simulink model "CalibrationMotorbike_v2"  (R2020b)
settings: Solver=FixedStepDiscrete  StartTime=0.0  StopTime=inf  FixedStep=0.01  RelTol=1e-3  EnableMultiTasking=on
undefined symbols (not defined in the file or in its folder): fdesignblkfcn, gcbh
libraries: dspstat3 x11, dsparch4 x3, simulink x2, dspswit3 x1
(part 2 of 2)

== system CalibrationMotorbike_v2/Butterworth2nd9 ==
  cutOff-Freq : Inport
  U(t) : Inport  Port=2
  samplingTime : Inport  Port=3
  Add : Sum  Inputs=+++
  Add1 : Sum  Inputs=+-
  Add2 : Sum
  Add3 : Sum  Inputs=+-+
  Add4 : Sum
  Add5 : Sum  Inputs=+++
  Divide : Product  Inputs=*/
  Divide1 : Product  Inputs=*/
  Gain : Gain  Gain=2
  Gain1 : Gain  Gain=sqrt(2)
  Gain2 : Gain  Gain=2
  Gain3 : Gain  Gain=-2
  Product{,1..5,7..9} (9 alike) : Product  RndMeth=Zero
  Unit Delay{,1,3..4} (4 alike) : UnitDelay  SampleTime=-1  HasFrameUpgradeWarning=on
  const : Constant  Value=2*pi
  const3 : Constant  Value=2
  Y(t) : Outport  VectorParamsAs1DForOutWhenUnconnected=off
  wires:
  U(t)/1 -> Product1/2, Unit Delay/1
  Product/1 -> Product1/1, Product3/1, Product2/1, Gain/1, Add3/3, Add5/3
  Unit Delay/1 -> Unit Delay1/1, Gain2/1
  Unit Delay1/1 -> Product3/2
  Product1/1 -> Add/1
  Product2/1 -> Add/2
  Product3/1 -> Add/3
  Add/1 -> Add1/1
  Divide/1 -> Unit Delay3/1, Y(t)/1
  Product4/1 -> Add3/1, Add5/1, Gain3/1
  Gain/1 -> Add2/1
  Unit Delay3/1 -> Product7/2, Unit Delay4/1
  Add2/1 -> Product7/1
  Gain1/1 -> Product8/1
  Product8/1 -> Add3/2, Add5/2
  Unit Delay4/1 -> Product9/2
  Add3/1 -> Product9/1
  Product9/1 -> Add4/2
  Product7/1 -> Add4/1
  Add4/1 -> Add1/2
  Add1/1 -> Divide/1
  Add5/1 -> Divide/2
  Gain2/1 -> Product2/2
  Gain3/1 -> Add2/2
  Product5/1 -> Product/1, Product/2, Product8/2
  const/1 -> Product5/1
  cutOff-Freq/1 -> Product5/2
  const3/1 -> Divide1/1
  samplingTime/1 -> Divide1/2
  Divide1/1 -> Gain1/1, Product4/2, Product4/1

== system CalibrationMotorbike_v2/Double-Click Button to set current folder ==

== system CalibrationMotorbike_v2/Simulink Function ==
  Gravity_2_RotMatrix : TriggerPort  TriggerType=function-call  IsSimulinkFunction=on  FunctionName=Gravity_2_RotMatrix  FunctionVisibility=scoped  VariantControl=(inherit)
  Gravity_2_RotMatrixMat : MATLAB Function  TreatAsAtomicUnit=on
  gravity : ArgIn  DisableCoverage=on  OutDataTypeStr=single  PortDimensions=4  ArgumentName=gravity
  rot_Matrix : ArgOut  DisableCoverage=on  OutDataTypeStr=single  PortDimensions=[3 3]  ArgumentName=rot_Matrix
  wires:
  gravity/1 -> Gravity_2_RotMatrixMat/1(gravity)
  Gravity_2_RotMatrixMat/1(A) -> rot_Matrix/1

== system CalibrationMotorbike_v2/SmartACCFilter1 ==
  ACC_In : Inport
  Moving Average2 : dspstat3/Moving Average  Method=Sliding window  ForgettingFactorPort=off  SpecifyWindowLength=on  WindowLength=40  ForgettingFactor=0.9  SimulateUsing=Code generation
  Moving Standard Deviation2 : dspstat3/Moving Standard Deviation  Method=Sliding window  ForgettingFactorPort=off  SpecifyWindowLength=on  WindowLength=40  ForgettingFactor=0.9  SimulateUsing=Code generation
      settings: SourceProductBaseCode=DS
  SmartFilter2 : MATLAB Function  TreatAsAtomicUnit=on
  accSf_mg_SmartFilter : Outport
  accSf_mg_SmartFilter_k : Outport  Port=2
  accSf_mg_Average20 : Outport  Port=3
  accSf_mg_Std20 : Outport  Port=4
  wires:
  SmartFilter2/2(k_out) -> accSf_mg_SmartFilter_k/1
  SmartFilter2/1(y_out) -> accSf_mg_SmartFilter/1
  Moving Average2/1 -> accSf_mg_Average20/1, SmartFilter2/1(x_mean)  "accSfXmg_Average20"
  Moving Standard Deviation2/1 -> SmartFilter2/2(x_std), accSf_mg_Std20/1
  ACC_In/1 -> Moving Average2/1, Moving Standard Deviation2/1

== system CalibrationMotorbike_v2/SmartACCFilter2 ==
  note: Smart Filtering depending on current noise/motion
      |
      | Low-Noise/Motion	-> fast signal following
      | High-Noise/Motion	-> high filtering (=slow following)
  ACC_In : Inport
  Moving Average2 : dspstat3/Moving Average  Method=Sliding window  ForgettingFactorPort=off  SpecifyWindowLength=on  WindowLength=40  ForgettingFactor=0.9  SimulateUsing=Code generation
  Moving Standard Deviation2 : dspstat3/Moving Standard Deviation  Method=Sliding window  ForgettingFactorPort=off  SpecifyWindowLength=on  WindowLength=40  ForgettingFactor=0.9  SimulateUsing=Code generation
      settings: SourceProductBaseCode=DS
  SmartFilter2 : MATLAB Function  TreatAsAtomicUnit=on
  accSf_mg_SmartFilter : Outport
  accSf_mg_SmartFilter_k : Outport  Port=2
  accSf_mg_Average20 : Outport  Port=3
  accSf_mg_Std20 : Outport  Port=4
  wires:
  ACC_In/1 -> Moving Standard Deviation2/1, Moving Average2/1
  Moving Standard Deviation2/1 -> accSf_mg_Std20/1, SmartFilter2/2(x_std)
  Moving Average2/1 -> SmartFilter2/1(x_mean), accSf_mg_Average20/1  "accSfXmg_Average20"
  SmartFilter2/1(y_out) -> accSf_mg_SmartFilter/1
  SmartFilter2/2(k_out) -> accSf_mg_SmartFilter_k/1

== system CalibrationMotorbike_v2/SmartACCFilter3 ==
  ACC_In : Inport
  Moving Average2 : dspstat3/Moving Average  Method=Sliding window  ForgettingFactorPort=off  SpecifyWindowLength=on  WindowLength=40  ForgettingFactor=0.9  SimulateUsing=Code generation
  Moving Standard Deviation2 : dspstat3/Moving Standard Deviation  Method=Sliding window  ForgettingFactorPort=off  SpecifyWindowLength=on  WindowLength=40  ForgettingFactor=0.9  SimulateUsing=Code generation
      settings: SourceProductBaseCode=DS
  SmartFilter2 : MATLAB Function  TreatAsAtomicUnit=on
  accSf_mg_SmartFilter : Outport
  accSf_mg_SmartFilter_k : Outport  Port=2
  accSf_mg_Average20 : Outport  Port=3
  accSf_mg_Std20 : Outport  Port=4
  wires:
  ACC_In/1 -> Moving Standard Deviation2/1, Moving Average2/1
  Moving Standard Deviation2/1 -> accSf_mg_Std20/1, SmartFilter2/2(x_std)
  Moving Average2/1 -> SmartFilter2/1(x_mean), accSf_mg_Average20/1  "accSfXmg_Average20"
  SmartFilter2/1(y_out) -> accSf_mg_SmartFilter/1
  SmartFilter2/2(k_out) -> accSf_mg_SmartFilter_k/1

== matlab function CalibrationMotorbike_v2/SmartACCFilter1/SmartFilter2 ==
  data: x_mean input; y_out output; x_std input; k_out output
function [y_out,k_out]= fcn(x_mean, x_std)
    persistent y;
    persistent k;

    k_max   =  5;
    k_min   =  0.001;
    k_filter =  0.001;
    std_min =  1000;
    std_max =  2000;
    
    % Initialisation of internal Buffers on Startup
    if isempty(y)        
            y = double(x_mean);
            k = k_max;
    end
    
    
    % Adapt k Lowpass in dependancy of Standard daviation (low noise = const. Riding = faster filter)      
    k_in = k_min;
    if (x_std<std_min)
        k_in = double(k_max);
    elseif (x_std<std_max)
        k_in = double( (((k_min-k_max)/(std_max-std_min))*(x_std-std_min)+k_max));
    else
        k_in = double(k_min);
    end

    % Smoothen k filter to avoid fast k-changes in small low-noise
    % sequences
    % if k is smaller/slower (due to noise in signal) always reduce k fast
    if (k_in > k)
        k = k_filter*k_in + (1-k_filter) * k;
    else
        k = k_in;
    end
    
    %lowpass of Rawdata
    y = double(((1000-k)*y + k * x_mean)/1000);

    k_out = k;
    y_out = y;
end

== matlab function CalibrationMotorbike_v2/SmartACCFilter2/SmartFilter2 ==
  data: x_mean input; y_out output; x_std input; k_out output
function [y_out,k_out]= fcn(x_mean, x_std)
    persistent y;
    persistent k;

    k_max   =  5;
    k_min   =  0.001;
    k_filter =  0.001;
    std_min =  1000;
    std_max =  2000;
    
    % Initialisation of internal Buffers on Startup
    if isempty(y)        
            y = double(x_mean);
            k = k_max;
    end
    
    
    % Adapt k Lowpass in dependancy of Standard daviation (low noise = const. Riding = faster filter)      
    k_in = k_min;
    if (x_std<std_min)
        k_in = double(k_max);
    elseif (x_std<std_max)
        k_in = double( (((k_min-k_max)/(std_max-std_min))*(x_std-std_min)+k_max));
    else
        k_in = double(k_min);
    end

    % Smoothen k filter to avoid fast k-changes in small low-noise
    % sequences
    % if k is smaller/slower (due to noise in signal) always reduce k fast
    if (k_in > k)
        k = k_filter*k_in + (1-k_filter) * k;
    else
        k = k_in;
    end
    
    %lowpass of Rawdata
    y = double(((1000-k)*y + k * x_mean)/1000);

    k_out = k;
    y_out = y;
end

== matlab function CalibrationMotorbike_v2/SmartACCFilter3/SmartFilter2 ==
  data: x_mean input; y_out output; x_std input; k_out output
function [y_out,k_out]= fcn(x_mean, x_std)
    persistent y;
    persistent k;

    k_max   =  5;
    k_min   =  0.001;
    k_filter =  0.001;
    std_min =  1000;
    std_max =  2000;
    
    % Initialisation of internal Buffers on Startup
    if isempty(y)        
            y = double(x_mean);
            k = k_max;
    end
    
    
    % Adapt k Lowpass in dependancy of Standard daviation (low noise = const. Riding = faster filter)      
    k_in = k_min;
    if (x_std<std_min)
        k_in = double(k_max);
    elseif (x_std<std_max)
        k_in = double( (((k_min-k_max)/(std_max-std_min))*(x_std-std_min)+k_max));
    else
        k_in = double(k_min);
    end

    % Smoothen k filter to avoid fast k-changes in small low-noise
    % sequences
    % if k is smaller/slower (due to noise in signal) always reduce k fast
    if (k_in > k)
        k = k_filter*k_in + (1-k_filter) * k;
    else
        k = k_in;
    end
    
    %lowpass of Rawdata
    y = double(((1000-k)*y + k * x_mean)/1000);

    k_out = k;
    y_out = y;
end

== matlab function CalibrationMotorbike_v2/MATLAB Function1 ==
  data: initRotMat input; init_valid output
function init_valid  = fcn(initRotMat)

  
    if sum(diag(initRotMat)) == 3 || sum(sum(initRotMat))== 0 %not calibrated yet (detect identity matrix or zero matrix)
        init_valid = 0;
    else    %inital calibration is existing
        init_valid = 1;
    end

== matlab function CalibrationMotorbike_v2/Rotate_to_Gravity ==
  data: x input; x_rot output; y input; z input; x_gravity input; y_gravity input; z_gravity input; y_rot output; z_rot output
% Rotates the input Signal depending on the gravity vector.
% As a Result the x,y,z will show in the always in the same direction
% (independant of mounting position or posture)
% The X-komponent from the Input will show towards the floor.


function [x_rot,y_rot, z_rot] = fcn(x, y, z, x_gravity, y_gravity, z_gravity)

	%Transformation Matrix ausrechnen mit gravity
	x_rot=x;
	y_rot=y;
	z_rot=z;

	a	= sqrt(x_gravity*x_gravity+y_gravity*y_gravity+z_gravity*z_gravity);
    
    if a~=0
			n1 = x_gravity/a+1;
			n2 = y_gravity/a;
			n3 = z_gravity/a;

			a	= sqrt(n1*n1+n2*n2+n3*n3);
			n1 = n1/a;
			n2 = n2/a;
			n3 = n3/a;


			x_rot = (n1*n1*2-1)	*(x)	+	(n1*n2*2)	*(y)	+ (n1*n3*2)		*(z);
			y_rot = (n2*n1*2)	*(x)	+	(n2*n2*2-1)	*(y)	+ (n2*n3*2)		*(z);
			z_rot = (n3*n1*2)	*(x)	+	(n3*n2*2)	*(y)	+ (n3*n3*2-1)	*(z);

    end

== matlab function CalibrationMotorbike_v2/Direction_Vector ==
  data: y input; abs output; z input; alpha output; alphastate output
function [abs,alpha,alphastate] = fcn(y, z)

persistent alpha_estimate;
persistent alpha_max;
persistent abs_max;

    % Initialisation of internal Buffers on Startup
    if isempty(alpha_estimate)        
            alpha_estimate = 0; 
            alpha_max =0;
            abs_max = 0;
    end    

abs = sqrt(y*y+z*z);

if abs>0
    alpha = atan2(y,z) * (180 / pi);
else
    alpha = 0;
end

%if z<0 
%    if y>=0  
%        alpha=alpha+180;
%    else
%        alpha=alpha-180;        
%    end
%end

if alpha < -180
    alpha=alpha+360;   
end

if alpha > 180
    alpha=alpha-360;   
end



% Maximum (Peak within Break/Accel)) should contain most reliebale aplha-Estimation
if abs > abs_max
    abs_max     = abs;
    alpha_max   = alpha;
else
    alpha_estimate = alpha;
    abs_max     = 0;
    alpha_max   = 0;
end
    

alphastate = alpha_estimate;

== matlab function CalibrationMotorbike_v2/MATLAB Function ==
  data: accel input; accel_rot output; gyro input
function accel_rot = fcn(accel,gyro)

persistent FUSE;

% GyroscopeNoise and AccelerometerNoise is determined from datasheet.
GyroscopeNoiseMPU9250       = 1e-06; % GyroscopeNoise (variance) in units of rad/s
AccelerometerNoiseMPU9250   = 0.1; % AccelerometerNoise (variance) in units of m/s^2


if isempty(FUSE)
    FUSE = imufilter('SampleRate', 0.01 , 'GyroscopeNoise',GyroscopeNoiseMPU9250,'AccelerometerNoise', AccelerometerNoiseMPU9250);
end


rotators = FUSE(accel',gyro');

%accel_rot = rotateframe(rotators,accel)

accel_rot = rotateframe(rotators,accel')

== matlab function CalibrationMotorbike_v2/Simulink Function/Gravity_2_RotMatrixMat ==
  data: gravity input; A output
% Rotates the input Signal depending on the gravity vector.
% As a Result the x,y,z will show in the always in the same direction
% (independant of mounting position or posture)
% The X-komponent from the Input will show towards the floor.
% -> e.g. if no movement or activity availible the result will be:
%		(x)		(1g)
%		(y)	->	(0)
%		(z)		(0)
%
% der Winkel zwischen zwei Vektoren aus dem Skalarprodukt:
% 	_   _
% 	x * y = |x|*|y|*cos(a(x,y)) = x1*y2 + x2*y2 + x3*y3
% 
% 			_   _
% 			x * y	  	x1*y2 + x2*y2 + x3*y3
% 	cos(a)=	------	= ------------------------
% 			|x|*|y|	sqrt((x1²+x2²+x3²)*(y1²+y2²+y3²))
% 
% der Vektor um den gedreht werden soll (Senskrecht zu Vektor a & b)
% 
% 	_   _	( x2*y3 - x3*y2 )	(v1)
% 	x x y = ( x3*y1 - x1*y3 ) =	(v2)
% 			( x1*y2 - x2*y1 )	(v3)
% 
% umformen zum Einheitsvektor:
% 			 _			_
% 		_	 v			v
% 		e = ---	= ---------------
% 			|v|	  sqrt(v1²+v2²+v3²) 			
% 
% Einsetzen in die allgemeine Rotationsmatrix http://de.wikipedia.org/wiki/Drehmatrix
% 
% oder über Eulerwinkel (Herleitung s. Schmierpapier)
% 
% 	x,y,z				=Gravitation	
% 	xx,yy,zz			=Rohsignal
% 	a=sqrt(x²+y²+z²)	=Betrag für Einheitsvektor
% 
% 	xcal= (sqrt((x*x+y*y)/(x*x+y*y))*(x*xx+z*zz)+y*yy)/a;
% 	ycal= (-x*y*xx-z*y*zz+(x*x+z*z)*yy)/(a*sqrt(x*x+z*z)) ;
% 	zcal= (-z*xx+x*zz)/sqrt(x*x+z*z);
% 
% 	ggf. kann Sensor mit sich selbst Kalibriet (a!=1g) werden:  
% 
% 	xcal= (sqrt((x*x+y*y)/(x*x+y*y))*(x*xx+z*zz)+y*yy)/1;
% 	ycal= (-x*y*xx-z*y*zz+(x*x+z*z)*yy)/(1*sqrt(x*x+z*z)) ;
% 	zcal= a*(-z*xx+x*zz)/sqrt(x*x+z*z);
% 
% 
% 
% 	Versuch 3:
% 
% 	Ziel: der Gravitationsvektor wird so rotiert das : 
% 			[grav] * [T]	=[1,0,0]	gesucht ist [T]
% 
% 		dann wird der Messvektor analog gedreht
% 			[acc] * [T] = [acc']
% 
% http://matheplanet.com/default3.html?call=viewtopic.php?topic=64323&ref=https%3A%2F%2Fwww.google.de%2F
% Vector-Macros von
% https://developer.apple.com/legacy/library/samplecode/glut/Listings/gle_vvector_h.html
% 
% 
% Householder-Matrix:
% 
% 			 1 0 0
% 	mit I=	 0 1 0			a,b = 2 Vektoren gleicher größe [a]*[a]T = [b]T * [b]    
% 			 0 0 1
% 
% 
% 		 a und b müssen gleiche Länge d.h. betrag Vektor haben
% 		hier ist
% 						| x | 					| sqrt(x²+y²+z²) |
% 					a = | y |		und		b =	|		0		 |  
% 			 			| z |					|		0		 |
% 
% 
% 
% 		---
% 		|		(I-((a-b)*(a-b)^T)
% 		|		------------------					wenn a!=b
% 	H= -|		((a-b)^T*a), 
% 		|
% 		|		I								wenn a=b
% 		---
% 
% 		für
% 		Ha = b und Hb = a
% 
% 
% ---------------------- Versuch 4
% 
% http://www.onlinemathe.de/forum/Vektor-in-R3-drehen-Richtungsaenderung
% viel einfacher als drehen: du spigelst an der Winkelhalbierenden zwischen u- achse und deinem Vektor. 
% die Wh ist einfach die Summe der 2 Einheitsvektoren, 
% dann wieder normieren und dann hast du x -> x+2<v,x> * vv= Einheitsvektor er Wh.
% 
% 
% http://matheplanet.com/default3.html?call=viewtopic.php?topic=36080&ref=https%3A%2F%2Fwww.google.de%2F
% Wenn du zwei gleichlange Vektoren  a und b hast, dann ist a+b eine Winkelhalbierende des von a und b augespannten Winkels.
% 
% um die Winkelhabierende um 180° drehen mit drehmatrix:
% https://de.wikipedia.org/wiki/Drehmatrix
% 
% sin(180)=0
% cos(180)=-1
% 
% 


function A  = fcn(gravity)
    A=single(eye(3)); 
    w=single(0);
%	x=accel(1);
%	y=accel(2);
%	z=accel(3);    

	%Transformation Matrix ausrechnen mit gravity
%	x_rot=x;
%	y_rot=y;
%	z_rot=z;

	a	= sqrt(gravity(1)*gravity(1)+gravity(2)*gravity(2)+gravity(3)*gravity(3));
    
    if a>10 % should be ~=0 but due to float-precision issues something close to 0 could be the output -> 1g =1000 so anything <10 is not valid
			n1 = gravity(1)/a+1;
			n2 = gravity(2)/a;
			n3 = gravity(3)/a;

			a	= sqrt(n1*n1+n2*n2+n3*n3);
			n1 = n1/a;
			n2 = n2/a;
			n3 = n3/a;

%			x_rot = (n1*n1*2-1)	*(x)	+	(n1*n2*2)	*(y)	+ (n1*n3*2)		*(z);
%			y_rot = (n2*n1*2)	*(x)	+	(n2*n2*2-1)	*(y)	+ (n2*n3*2)		*(z);
%			z_rot = (n3*n1*2)	*(x)	+	(n3*n2*2)	*(y)	+ (n3*n3*2-1)	*(z);

% Transform Rot-Matrix to Bosch.IO format (Z = GroundVector -> toggle X,Z) 

            A(3,1) = (n1*n1*2-1);
            A(3,2) = (n1*n2*2);
            A(3,3) = (n1*n3*2);

            A(2,1) = (n2*n1*2);
            A(2,2) = (n2*n2*2-1);
            A(2,3) = (n2*n3*2);

            A(1,1) = (n3*n1*2); 
            A(1,2) = (n3*n2*2);
            A(1,3) = (n3*n3*2-1);
            
            
            %Angle rotation
            w = gravity(4);
        %    w = -w;
            if (w ~=0 )
                w = w * pi/180;
        %        y_rot2 = cos(w) * y_rot- sin(w) * z_rot;
        %        z_rot2 = sin(w) * y_rot+ cos(w) * z_rot;
                A_temp = A;

                A(2,1) = -cos(w) * A_temp(2,1) + sin(w) * A_temp(1,1);
                A(2,2) = -cos(w) * A_temp(2,2) + sin(w) * A_temp(1,2);
                A(2,3) = -cos(w) * A_temp(2,3) + sin(w) * A_temp(1,3);

                A(1,1) = sin(w) * A_temp(2,1) + cos(w) * A_temp(1,1);
                A(1,2) = sin(w) * A_temp(2,2) + cos(w) * A_temp(1,2);
                A(1,3) = sin(w) * A_temp(2,3) + cos(w) * A_temp(1,3);
            else
        %       y_rot2 = y_rot;
        %        z_rot2 = z_rot;
            end            
    end


  
    
% Transform Rot-Matrix to Bosch.IO format (Z = GroundVector)
%         A_temp = A
% 
%         A(1,1) = A_temp(3,1);
%         A(1,2) = A_temp(3,2);
%         A(1,3) = A_temp(3,3);
% 
%         A(2,1) = -A_temp(2,1);
%         A(2,2) = -A_temp(2,2);
%         A(2,3) = -A_temp(2,3);
% 
%         A(3,1) = A_temp(1,1);
%         A(3,2) = A_temp(1,2);
%         A(3,3) = A_temp(1,3);

== stateflow chart CalibrationMotorbike_v2/CalibrationState ==
  state ENGINE_STATE_ESTIMATOR [parallel]
    settings: executionOrder=1
    note: based on Vibration (Variance in ACC)
    state ENGINE_OFF
      state_Ignition=0;
    state ENGINE_ON
    note: to avoid ignition=true in case of variance caused by motion (e.g. tilting, Walking)
        | engine causes constant vibration
    (default) -> ENGINE_OFF
    ENGINE_OFF -> ENGINE_STATE_ESTIMATOR.ENGINE_ON : [accSfmg_Variance>4000]
    ENGINE_STATE_ESTIMATOR.ENGINE_ON -> ENGINE_OFF [order 1] : [accSfmg_Variance<1000]
    ENGINE_STATE_ESTIMATOR.ENGINE_ON -> ENGINE_STATE_ESTIMATOR.ENGINE_ON [order 2] : [after(10,sec) || ...
        | speed_kmh>5]
        | {state_Ignition=1;}
  state ACCELERATION_STATE_ESTIMATOR [parallel]
    settings: executionOrder=2
    note: (Stationary, Accel, Break) based on normalized Acceleration Signal
    state INIT_DIRECTION
      state_Acceleration = 0;
      rough_direction_angle_fwd=-1;
    state DIRECTION_FOUND_ACCEL
      if (abs(Direction_alpha) < 90)
      Break_equals_Negative=1;
      else
      Break_equals_Negative=0;
      end;
      rough_direction_angle_fwd=Direction_alpha;
    state DIRECTION_FOUND_BREAK
      if (abs(Direction_alpha) < 90)
      Break_equals_Negative=0;
      else
      Break_equals_Negative=1;
      end;
      rough_direction_angle_fwd=Direction_alpha+180;
      if (rough_direction_angle_fwd>360)
      rough_direction_angle_fwd = rough_direction_angle_fwd-360;
      end
    note: Init to detect Phone Display-Direction
        | (Display showing forward or backward)
        | (usually to driver but it might be different)
    state STATIONARY
      state_Acceleration = 4;
    state ACCELERATION_POSITIVE
      state_Acceleration = 5;
    state ACCELERATION_NEGATIVE
      state_Acceleration = 3;
    note: Stay in Accel/Break until normalized Accel small or
        | direction angle toggles negativ <-> positive direction
    (default) -> INIT_DIRECTION
    INIT_DIRECTION -> (junction 204) : [accFiltSfNorm > 200 && state_Direction>1 && ...
        | ((state_Riding==5) || (state_Riding==3))]
    (junction 204) -> DIRECTION_FOUND_ACCEL [order 1] : [state_Riding==5]
    (junction 204) -> DIRECTION_FOUND_BREAK [order 2]
    DIRECTION_FOUND_BREAK -> STATIONARY
    DIRECTION_FOUND_ACCEL -> STATIONARY
    ACCELERATION_NEGATIVE -> STATIONARY : [accFiltSfNorm < 175 || ...
        | abs(angle_diff(Direction_alpha,rough_direction_angle_fwd)) < 90]
    ACCELERATION_POSITIVE -> STATIONARY : [accFiltSfNorm < 175 ||...
        | abs(angle_diff(Direction_alpha,rough_direction_angle_fwd)) > 90]
    STATIONARY -> (junction 191) : [accFiltSfNorm > 300]
    (junction 191) -> ACCELERATION_POSITIVE [order 1] : [abs(angle_diff(Direction_alpha,rough_direction_angle_fwd)) < 90]
    (junction 191) -> ACCELERATION_NEGATIVE [order 2] : %else
  state CALIBRATION_STATE_ESTIMATOR [parallel]
    settings: executionOrder=6
    state IDLE1
      state_Calibration=0;
      update_Calibration(0);
    state ENGINE_ON
      state UNKNOWN_DRIVING
        if (state_Curve==0)
        state_Calibration=0;
        else
        state_Calibration=-1;
        end;
        update_Calibration(0);
      state DRIVING_IN_DIRECTION_BREAK
        state_Calibration=30;
        GravityBreaking= ...
        update_GravVector( ...
        GravityBreaking);
        update_Calibration(state_Calibration);
      state DRIVING_OUT_DIRECTION_ACCEL
        state_Calibration=50;
        GravityAccel= ...
        update_GravVector( ...
        GravityAccel);
        update_Calibration(state_Calibration);
      state STANDING_STILL
        state_Calibration=10;
        GravityStanding= ...
        update_GravVector( ...
        GravityStanding);
        update_Calibration(state_Calibration);
      state STRAIGHT_DRIVING
        state_Calibration=40;
        GravityRiding= ...
        update_GravVector( ...
        GravityRiding);
        update_Calibration(state_Calibration);
      (default) -> UNKNOWN_DRIVING
      (junction 216) -> (junction 122)
      UNKNOWN_DRIVING -> (junction 122)
      (junction 122) -> UNKNOWN_DRIVING [order 5]
      (junction 122) -> STANDING_STILL [order 1] : [state_Riding==0 && ...
          | accSfmg_Variance<200000 && ...
          | state_Curve==0]
      (junction 122) -> DRIVING_OUT_DIRECTION_ACCEL [order 4] : [state_Riding==5 && ...
          | (state_Acceleration==5 || state_Direction == 3) && ...
          | state_Curve == 0 && ...
          | state_Direction > 1]
      (junction 122) -> DRIVING_IN_DIRECTION_BREAK [order 3] : [state_Riding==3 && ...
          | (state_Acceleration==3 || state_Direction == 3)&& ...
          | state_Curve == 0 && ...
          | state_Direction > 1]
      (junction 122) -> STRAIGHT_DRIVING [order 2] : [state_Riding==4 && ...
          | state_Curve==0]
      DRIVING_IN_DIRECTION_BREAK -> (junction 216)
      DRIVING_OUT_DIRECTION_ACCEL -> (junction 216)
      STRAIGHT_DRIVING -> (junction 216)
      STANDING_STILL -> (junction 216)
    (default) -> IDLE1 : {
        | state_Ignition=0;
        | state_Acceleration=0;
        | state_Riding=0;
        | state_Curve=0;
        | state_Direction=0;
        | state_Calibration=0;
        | GravityStanding =0* Gravity;
        | GravityRiding   = 0*Gravity;
        | GravityBreaking =0*Gravity;
        | GravityAccel =0*Gravity;
        | Calibration_Vector =0*Gravity;
        | calibrationOUT =zeros(12, 1);
        | }
    CALIBRATION_STATE_ESTIMATOR.ENGINE_ON -> IDLE1 : [state_Ignition==0]
    IDLE1 -> CALIBRATION_STATE_ESTIMATOR.ENGINE_ON : [state_Ignition>0]
  state RIDING_STATE_ESTIMATION [parallel]
    settings: executionOrder=3
    note: RIDING_State (Driving, Accel, Breaking etc.) based on current Speed (via GPS)
    state STANDING
      state_Riding=0;
    state RIDING_SLOW
      state_Riding=1;
    state RIDING
      note: Speed-Update depends on GPS (react on Change in "check or latest after x=2 sec)
      state RIDING_CONST
        state_Riding=4;
        speed_kmh_prev = speed_kmh;
      state RIDING_CONST_check
        speed_kmh_prev_n2 = speed_kmh_prev;
      state RIDING_DECELERATION
        entry:
        speed_kmh_prev = speed_kmh;
      state RIDING_ACCELERATION
        entry:
        speed_kmh_prev = speed_kmh;
      state RIDING_ACCELERATION_check
      state RIDING_DECELERATION_check
      (default) -> RIDING_CONST
      RIDING_DECELERATION_check -> RIDING_CONST [order 1] : [speed_kmh >= speed_kmh_prev-0.25]
      RIDING_ACCELERATION_check -> RIDING_CONST [order 1] : [speed_kmh <= speed_kmh_prev+0.25]
      RIDING_CONST_check -> RIDING_CONST [order 3]
      RIDING_CONST -> RIDING_CONST_check : [after(2,sec) || ...
          | speed_kmh ~= speed_kmh_prev]
      RIDING_CONST_check -> RIDING_ACCELERATION [order 2] : [speed_kmh > min(speed_kmh_prev,speed_kmh_prev_n2)+2]
      RIDING_CONST_check -> RIDING_DECELERATION [order 1] : [speed_kmh < max(speed_kmh_prev,speed_kmh_prev_n2)-2]
      RIDING_ACCELERATION_check -> RIDING_ACCELERATION [order 2] : {state_Riding=5;}
      RIDING_DECELERATION_check -> RIDING_DECELERATION [order 2] : {state_Riding=3;}
      RIDING_ACCELERATION -> RIDING_ACCELERATION_check : [after(2,sec) || ...
          | speed_kmh ~= speed_kmh_prev]
      RIDING_DECELERATION -> RIDING_DECELERATION_check : [after(2,sec) || ...
          | speed_kmh ~= speed_kmh_prev]
    (default) -> STANDING : {speed_kmh_prev=single(0);
        | speed_kmh_prev_n2=single(0);}
    RIDING_SLOW -> RIDING [order 1] : [speed_kmh>15]
    STANDING -> RIDING_SLOW : [speed_kmh>5]
    RIDING -> RIDING_SLOW : [speed_kmh<7]
    RIDING_SLOW -> STANDING [order 2] : [speed_kmh<3]
  state CURVE_STATE_ESTIMATION [parallel]
    settings: executionOrder=4
    note: based on integration of Gyro (via mean of moving window)
    state STRAIGHT
      state_Curve=0;
    state CURVE
      state_Curve=1;
    (default) -> STRAIGHT
    CURVE -> STRAIGHT : [gyrSfmdegs_FiltAverage<4000]
    STRAIGHT -> CURVE : [gyrSfmdegs_FiltAverage>6000]
  state STABLEDIRECTION_STATE_ESTIMATION [parallel]
    settings: executionOrder=5
    note: based on Driving (caused by Accleration and Breaking)
        | only stable (=const) Angles will be considred for calibration
    state UNKNOWN_DIRECTION
      state_Direction=0;
    note: Either Strong Direction-Signal or Stable Direction
    state KNOWN_DIRECTION
      state_Direction=1;
    state STABLE_DIRECTION
      state_Direction=2;
    note: only longer break/accel
        | periods have a stable angle
    note: very long break/accel period
        | so angle is very reliable
    state TRUSTABLE_DIRECTION
      state_Direction=3;
    (default) -> UNKNOWN_DIRECTION
    TRUSTABLE_DIRECTION -> UNKNOWN_DIRECTION : [Direction_alpha_Variance>5]
    STABLE_DIRECTION -> UNKNOWN_DIRECTION [order 2] : [(Direction_alpha_Variance>10+10 || ...
        |    Direction_absAverage < 100-60)]
    KNOWN_DIRECTION -> UNKNOWN_DIRECTION [order 1] : [(Direction_alpha_Variance>10+5 || ...
        |    Direction_absAverage < 100-50)]
    UNKNOWN_DIRECTION -> KNOWN_DIRECTION : [(Direction_alpha_Variance<10 && ...
        | Direction_absAverage > 100)]
    KNOWN_DIRECTION -> STABLE_DIRECTION [order 2] : [after(1,sec)]
    STABLE_DIRECTION -> TRUSTABLE_DIRECTION [order 1] : [after(2,sec) && Direction_alpha_Variance<1]
  data: alpha function_input; beta function_input; diff function_output; acc function_input; acc_out function_output; state_now function_input; calibrationOUT output; state_Calibration output size=1; Calibration_Vector output; state_Ignition output; speed_kmh input; accSfmg_Variance input; accFiltSfNorm input; gyrSfmdegs_FiltAverage input; Direction_absAverage input; Direction_alpha_Variance input; Direction_alpha input; state_Riding output; state_Acceleration output; state_Curve output; speed_kmh_prev local; state_Direction output; Gravity input; GravityStanding output; GravityRiding output; GravityBreaking output; Break_equals_Negative local; GravityAccel output; speed_kmh_prev_n2 local; rough_direction_angle_fwd local
  function diff = angle_diff(alpha,beta):
    | function diff = angle_diff(alpha,beta)
    | 
    | diff = alpha-beta;
    | if diff>180
    |     diff = diff -360;
    | end
    | 
    | if diff<-180
    |     diff = diff +360;
    | end
    | 
    | 
    | end
  function acc_out  = update_GravVector(acc):
    | function acc_out  = update_GravVector(acc)
    | 
    |     acc_out = acc;    
    |     n       = acc(5);  %number of Cycle updated
    |     
    |     alpha   = Direction_alpha;
    |     
    |     %Calibrate Axis depending on Screen-Orientation
    |     %if (Break_equals_Negative == 1)
    | %        alpha   = Direction_alpha;
    | %    else
    | %        alpha   = Direction_alpha+180;
    | %        if (alpha>180)
    | %            alpha = alpha -360;
    | %        end
    | %    end
    | 
    | 
    | 
    |     %Alpha might show forward backward depending on break/accel
    |     % Calibration-Alpha should always show forward 
    |     % if heading backward -> rotate 180°
    |     %if (alpha>90)        
    | %        alpha = alpha -180;
    | %    elseif (alpha < -90)
    | %        alpha = alpha +180;
    | %    end
    |     
    |       
    |     diff = alpha-rough_direction_angle_fwd;
    |     if diff>180
    |         diff = diff -360;
    |     end
    | 
    |     if diff<-180
    |         diff = diff +360;
    |     end
    |  
    |     if (abs(diff)>90) %most likelly breaking -> invert angle
    |         alpha = alpha +180;
    |         if alpha>180
    |            alpha = alpha -360;
    |         end
    |     end
    |     
    |     
    |     k_now = 0.0001;
    |     
    |     %Increase filter Speed during Initialization
    |     if (n <= 0)
    |         k_now=1;
    |     elseif (n < 10)
    |         k_now = 0.1;
    |     elseif (n < 30)
    |         k_now = 0.05;
    |     elseif (n < 100)
    |         k_now = 0.02;        
    |     else 
    |         k_now = 0.01;
    |     end
    |     
    |     if (k_now > 1) 
    |         k_now =1;
    |     end
    | 
    |     
    |     acc_out(1) = k_now * Gravity(1) + (1-k_now) * acc(1);
    |     acc_out(2) = k_now * Gravity(2) + (1-k_now) * acc(2);
    |     acc_out(3) = k_now * Gravity(3) + (1-k_now) * acc(3);
    |     if state_Direction > 1 %Update Direction Angle only if useful
    |         acc_out(4) = k_now * alpha     + (1-k_now) * acc(4);       
    |     end
    |     
    |    
    |     
    |     if acc(5)<100000 %avoid overflow
    |       acc_out(5) = n + 1;
    |     end
  function update_Calibration(state_now):
    | 
    | %Update the calibration vector based on current situation and state of
    | %Calibration
    | function update_Calibration(state_now)
    | 
    | persistent calibration;
    | 
    |     %Initialize Calibration internal values
    |     if isempty(calibration)        
    |         calibration.state      = 0; %start=0, init=1 (1st iniitilization phase), find =2 (fast finding of calibration), optimize =3 (optimize calibration estimation), hold=4 (done -> calibration known only minor updates)
    |         calibration.n          = 0;
    |         calibration.n_standing = 0;
    |         calibration.n_riding   = 0;
    |         calibration.n_breaking = 0;
    |         calibration.n_acclerating = 0;
    |         calibration.n_block    = 0;
    |         calibration.last_state = 0;
    |         calibration.blockCnt_standing = 0;
    |         calibration.blockCnt_riding   = 0;
    |         calibration.blockCnt_breaking = 0;
    |         calibration.blockCnt_acclerating = 0;
    | 
    |     end
    |     
    | 
    |     if (calibration.state == 0)         % Initialization -> use Gravity Vectror as best guess (e.g. to initilize following filters and to avoid a signal jump at 1st Calibration-Vector estimation)
    |         Calibration_Vector(1)  = Gravity(1);
    |         Calibration_Vector(2)  = Gravity(2);
    |         Calibration_Vector(3)  = Gravity(3);        
    |         Calibration_Vector(4)  = 0;
    |     end
    | 
    |     %start new block if state toogles (e.g. from "unknown" to Standing)
    |     if (calibration.last_state ~= state_now)
    |          calibration.n_block    = 0;
    |     end
    |     
    |     
    | 
    |     k = 1;
    |     k2 = 1;
    |     % Update Vector (different actions depending on kind of situation)            
    |     % **********************************************************    
    |     % ******************************* Standing State ***********    
    |     if state_now == 10      % Standing State        
    |         % -> indication of Gravity (no noise but with Errors due to possible tilting during Stand, no Direction)        
    |         
    |         if (calibration.state == 0)         % 1st sample Initialization -> use any 1st value as start
    |             k = 1;          
    |         elseif (calibration.state == 1)     % initphase =1 iniitilization phase -> fast update
    |             k = 0.1;  
    |         elseif (calibration.state == 2)     % findphase =2 (fast finding of calibration)
    |             k = 0.01;
    |         else                                % 3/4 ignore Standing-Calibration as soon as enough updates availible
    |             k = 0;
    |         end
    |         
    |         Calibration_Vector(1)  = k * GravityStanding(1) + (1-k) * Calibration_Vector(1);
    |         Calibration_Vector(2)  = k * GravityStanding(2) + (1-k) * Calibration_Vector(2);
    |         Calibration_Vector(3)  = k * GravityStanding(3) + (1-k) * Calibration_Vector(3);        
    |         Calibration_Vector(4)  = k * GravityBreaking(4) + (1-k) * Calibration_Vector(4);        
    |         if (calibration.n_standing<1000000) 
    |             calibration.n_standing = calibration.n_standing+1;
    |         end
    |         if (k>0 && calibration.n<1000) %ignore cnt>1000  in Standing State
    |             calibration.n = calibration.n+1;
    |         end        
    |         if (calibration.n_block == 0 && calibration.blockCnt_standing<1000000) 
    |             calibration.blockCnt_standing = calibration.blockCnt_standing+1;
    |         end        
    |     % *****************************************************************    
    |     % ******************************* Straight Riding State ***********    
    |     elseif state_now == 40   %
    |         % -> indication of Gravity (only with noise due to Motion of Riding, poor Direction-Estimation)
    | 
    |         if (calibration.state == 0)         %1st Initialization -> use any 1st value as start
    |             k = 1;          
    |             k2 = k;          
    |         elseif (calibration.state == 1)     % initphase =1 iniitilization phase -> fast update
    |             k = 0.1;  
    |             k2 = k;  
    |         elseif (calibration.state == 2)     % findphase =2 (fast finding of calibration)
    |             k = 0.05;
    |             k2 = k;
    |         elseif (calibration.state == 3)     % optimize phase =3 (optimize calibration estimation)
    |             k = 0.01;
    |             if calibration.blockCnt_breaking<3
    |                 k2 =k;
    |             else %ignore angle during ride as soon as enough updates from breaking availible
    |                 k2 = 0;
    |             end
    |         else                                % hold phase =4 calibration done -> only minor updates
    |             %ignore during Ride update only hold caibration vector
    |             k = 0;
    |             k2 = k;
    |         end
    |         
    |                
    |         Calibration_Vector(1)  = k * GravityRiding(1) + (1-k) * Calibration_Vector(1);
    |         Calibration_Vector(2)  = k * GravityRiding(2) + (1-k) * Calibration_Vector(2);
    |         Calibration_Vector(3)  = k * GravityRiding(3) + (1-k) * Calibration_Vector(3);
    |         Calibration_Vector(4)  = k2 * GravityRiding(4) + (1-k2) * Calibration_Vector(4);
    |         Calibration_Vector(5)  = Calibration_Vector(5)+1;
    |         
    |         if (calibration.n_riding<1000000) 
    |             calibration.n_riding = calibration.n_riding+1;
    |         end
    |         if (k>0 && calibration.n<2000) %ignore cnt>1000  in Riding State
    |             calibration.n = calibration.n+1;
    |         end           
    |         if (calibration.n_block == 0 && calibration.blockCnt_riding<1000000) 
    |             calibration.blockCnt_riding = calibration.blockCnt_riding+1;
    |         end        
    |     % *****************************************************************    
    |     % ******************************* Breaking State ***********         
    |     elseif state_now == 30 % Breaking State         
    |         % -> indication of Direction-Angle (poor/no Gravity due to Breaking Maneuver but good Direction of Driving
    |         k = 0.0001;
    |         
    |         if (calibration.state == 0)         %1st Initialization -> use any 1st value as start
    |             k = 1;          
    |             k2 = k;          
    |         elseif (calibration.state == 1)     % initphase =1 iniitilization phase -> fast update
    |             k = 0.1;  
    |             k2 = k;  
    |             if (calibration.blockCnt_breaking <2) 
    |                 k2 =0.1;
    |             end
    |         elseif (calibration.state == 2)    % findphase =2 (fast finding of calibration)
    |             k = 0.05;
    |             k2 = k;
    |             if (calibration.blockCnt_breaking <2)
    |                 k2 =0.1;
    |             end
    |         elseif (calibration.state == 3)   % optimize phase =3 (optimize calibration estimation)
    |             k = 0.01;
    |             k2 =k;
    |             if (calibration.blockCnt_breaking <2) 
    |                 k2 =0.1;
    |             end
    |         else                                % hold phase =4 calibration done -> only minor updates
    |             %very slow update almost hold caibration vector
    |             k = 0.01;
    |             k2 = k;
    |             if (calibration.blockCnt_breaking <2) 
    |                 k2 =0.1;
    |             end
    |         end
    |         
    |         
    |         Calibration_Vector(1)  = k * GravityBreaking(1) + (1-k) * Calibration_Vector(1);
    |         Calibration_Vector(2)  = k * GravityBreaking(2) + (1-k) * Calibration_Vector(2);
    |         Calibration_Vector(3)  = k * GravityBreaking(3) + (1-k) * Calibration_Vector(3);        
    |         Calibration_Vector(4)  = k2 * GravityBreaking(4) + (1-k2) * Calibration_Vector(4);
    |         Calibration_Vector(5)  = Calibration_Vector(5)+1;
    |         if (calibration.n_breaking<1000000) 
    |             calibration.n_breaking = calibration.n_breaking+1;
    |         end
    |         if (k>0 && calibration.n<1000000) 
    |             calibration.n = calibration.n+1;
    |         end           
    |         if (calibration.n_block == 0 && calibration.blockCnt_breaking<1000000) 
    |             calibration.blockCnt_breaking = calibration.blockCnt_breaking+1;
    |         end        
    |     % *****************************************************************    
    |     % ******************************* Accelerating State ***********         
    |     elseif state_now == 50 % Accelerating State         
    |         % -> indication of Direction-Angle (poor/no Gravity due to Breaking Maneuver but good Direction of Driving
    |         k = 0.0001;
    |         
    |         if (calibration.state == 0)         %1st Initialization -> use any 1st value as start
    |             k = 1;          
    |             k2 = k;          
    |         elseif (calibration.state == 1)     % initphase =1 iniitilization phase -> fast update
    |             k = 0.1;  
    |             k2 = k;  
    |             if (calibration.blockCnt_acclerating <2) 
    |                 k2 =0.1;
    |             end
    |         elseif (calibration.state == 2)    % findphase =2 (fast finding of calibration)
    |             k = 0.05;
    |             k2 = k;
    |             if (calibration.blockCnt_acclerating <2)
    |                 k2 =0.1;
    |             end
    |         elseif (calibration.state == 3)   % optimize phase =3 (optimize calibration estimation)
    |             k = 0.01;
    |             k2 =k;
    |             if (calibration.blockCnt_acclerating <2) 
    |                 k2 =0.1;
    |             end
    |         else                                % hold phase =4 calibration done -> only minor updates
    |             %very slow update almost hold caibration vector
    |             k = 0.01;
    |             k2 = k;
    |             if (calibration.blockCnt_acclerating <2) 
    |                 k2 =0.1;
    |             end
    |         end
    |                 
    |         Calibration_Vector(1)  = k * GravityBreaking(1) + (1-k) * Calibration_Vector(1);
    |         Calibration_Vector(2)  = k * GravityBreaking(2) + (1-k) * Calibration_Vector(2);
    |         Calibration_Vector(3)  = k * GravityBreaking(3) + (1-k) * Calibration_Vector(3);        
    |         Calibration_Vector(4)  = k2 * GravityBreaking(4) + (1-k2) * Calibration_Vector(4);
    |         Calibration_Vector(5)  = Calibration_Vector(5)+1;
    |         if (calibration.n_acclerating<1000000) 
    |             calibration.n_acclerating = calibration.n_acclerating+1;
    |         end
    |         if (k>0 && calibration.n<1000000) 
    |             calibration.n = calibration.n+1;
    |         end           
    |         if (calibration.n_block == 0 && calibration.blockCnt_acclerating<1000000) 
    |             calibration.blockCnt_acclerating = calibration.blockCnt_acclerating+1;
    |         end                        
    |     else % Unknown State (and iginition on) -> no Calibration info availible        
    |         k =0;
    |     end
    |     
    |     
    | %Plausibility Check of Calibration
    |     %abs = sqrt(Calibration_Vector(1)*Calibration_Vector(1)+Calibration_Vector(2)*Calibration_Vector(2)+Calibration_Vector(3)*Calibration_Vector(3));        
    |     
    |     % Check if sufficient blocks availible to swithc to next calibrationmode/state
    |     if (calibration.state == 0)                         %0: 1st Initialization -> use any 1st value as start
    |         if (calibration.n>100)   %1st values availible
    |             calibration.state =1;
    |         end
    |     elseif (calibration.state == 1)                     %1: iniitilization phase -> fast update to get initial estimation
    |         if ((calibration.n>150) && (speed_kmh>3))        %init Phase done
    |             calibration.state =2;
    |         end
    |     elseif (calibration.state == 2)                     %2: findphase =2 -> fast finding of calibration
    |         if ((calibration.blockCnt_breaking >= 1) || (calibration.blockCnt_acclerating>=1)) &&  (calibration.blockCnt_riding>=1) %should have seen riding && (breaking or accel) at least once
    |             calibration.state =3;
    |         end
    |     elseif (calibration.state == 3)                     %3: optimize phase =3 (optimize calibration estimation)
    |         if ((calibration.blockCnt_breaking >= 1) && (calibration.blockCnt_acclerating >= 1) )  %should have seen all states at least once
    |             calibration.state =4;
    |         end
    |     else                                                %4: hold phase =4 calibration done -> only minor updates
    |     end
    |     
    |     
    |     
    |     
    |     %prepare for next cycle
    |     calibration.last_state = state_now;
    |     if (calibration.n_block<1000000) 
    |         calibration.n_block = calibration.n_block+1;
    |     end           
    |     
    |     
    |         calibrationOUT(1) = calibration.state      ;
    |         calibrationOUT(2) = calibration.n         ;
    |         calibrationOUT(3) = calibration.n_standing ;
    |         calibrationOUT(4) = calibration.n_riding   ;
    |         calibrationOUT(5) = calibration.n_breaking ;
    |         calibrationOUT(6) = calibration.n_acclerating ;        
    |         calibrationOUT(7) = calibration.n_block    ;
    |         calibrationOUT(8) = calibration.last_state ;
    |         calibrationOUT(9) = calibration.blockCnt_standing ;
    |         calibrationOUT(10) = calibration.blockCnt_riding   ;
    |         calibrationOUT(11) = calibration.blockCnt_breaking ;
    |         calibrationOUT(12) = calibration.blockCnt_acclerating ;
